simulink model "ISC_laboratorio_02_ex2"  (R2019a)
settings: Solver=VariableStepAuto  StartTime=0.0  StopTime=10.0  RelTol=1e-3
settings Model: Creator=guilh  LastModifiedBy=guilh

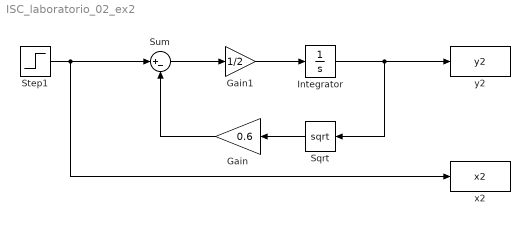
== system ISC_laboratorio_02_ex2 ==
  Gain : Gain  Gain=0.6
  Gain1 : Gain  Gain=1/2
  Integrator : Integrator  InitialCondition=1
  Sqrt : Sqrt  SaturateOnIntegerOverflow=on
  Step1 : Step  Time=0  Before=2  After=0  SampleTime=0
  Sum : Sum  Inputs=|+-
  x2 : ToWorkspace  VariableName=x2  SampleTime=-1
  "y2 " : ToWorkspace  VariableName=y2  SampleTime=-1
  wires:
  Integrator/1 -> Sqrt/1, "y2 "/1
  Sum/1 -> Gain1/1
  Step1/1 -> Sum/1, x2/1
  Gain/1 -> Sum/2
  Sqrt/1 -> Gain/1
  Gain1/1 -> Integrator/1
